simulink model "PID_controller"  (R2013a)
settings: Solver=ode45  StartTime=0.0  StopTime=10.0  RelTol=1e-3
settings Model: Creator=training-it  LastModifiedBy=Pera
settings DataIOCC: SignalLoggingSaveFormat=ModelDataLogs
settings DebuggingCC: MultiTaskDSMMsg=warning  MultiTaskCondExecSysMsg=none  StateNameClashWarn=none  StrictBusMsg=None
settings RTWCC: IncludeERTFirstTime=on

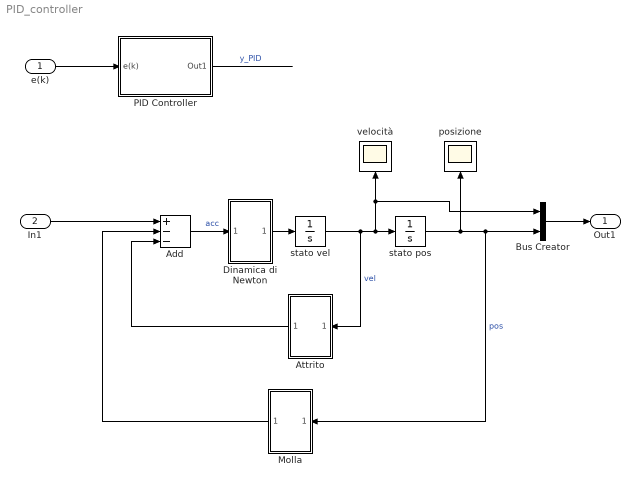
== system PID_controller ==
  e(k) : Inport
  In1 : Inport  Port=2
  Add : Sum  Inputs=+--
  Attrito : Subsystem  mask{c=2}
      mask prompts: c "coeff attrito"
  Bus Creator : BusCreator  Inputs=2
  Dinamica di Newton : Subsystem  mask{m=2}
      mask prompts: m "mass"
  Molla : Subsystem  mask{k=100}
      mask prompts: k "coeff elastico"
  PID Controller : Subsystem  mask{Ts=0.01, kp=0.3, ki=2, kd=0.1}
      mask prompts: Ts "Sample Time"; kp "Guadagno Proporzionale"; ki "Guadagno Integrativo"; kd "Guadagno Derivativo"
      mask init:
      | s1=['kp= ',num2str(kp)];
      | s2=['ki= ',num2str(ki)];
      | s3=['kd= ',num2str(ki)];
      | s=strvcat(s1,s2,s3);  %sto concatenando verticalmente
      mask Display: disp(s)
  posizione : Scope
  stato pos : Integrator  InitialCondition=x0  mask{x0=0}
      mask prompts: x0 "posizione iniziale"
  stato vel : Integrator  mask{v0=0}
      mask prompts: v0 "velocità iniziale"
  velocità : Scope
  Out1 : Outport
  wires:
  e(k)/1 -> PID Controller/1(e(k))
  PID Controller/1(Out1) -> ?  "y_PID"
  stato pos/1 -> Bus Creator/2, Molla/1(In1), posizione/1  "pos"
  Attrito/1(Out1) -> Add/3
  Molla/1(Out1) -> Add/2
  In1/1 -> Add/1
  Add/1 -> Dinamica di Newton/1(In1)  "acc"
  stato vel/1 -> Attrito/1(In1), velocità/1, Bus Creator/1, stato pos/1  "vel"
  Dinamica di Newton/1(Out1) -> stato vel/1
  Bus Creator/1 -> Out1/1

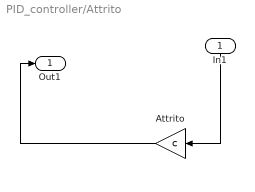
== system PID_controller/Attrito ==
  In1 : Inport
  Attrito : Gain  Gain=c
  Out1 : Outport
  wires:
  Attrito/1 -> Out1/1
  In1/1 -> Attrito/1

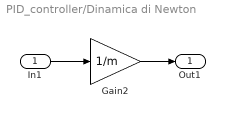
== system PID_controller/Dinamica di Newton ==
  In1 : Inport
  Gain2 : Gain  Gain=1/m
  Out1 : Outport
  wires:
  Gain2/1 -> Out1/1
  In1/1 -> Gain2/1

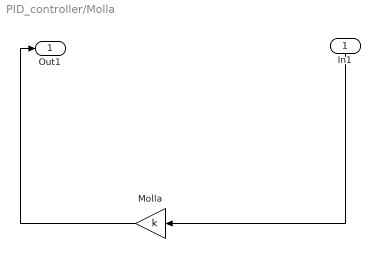
== system PID_controller/Molla ==
  In1 : Inport
  Molla : Gain  Gain=k
  Out1 : Outport
  wires:
  Molla/1 -> Out1/1
  In1/1 -> Molla/1

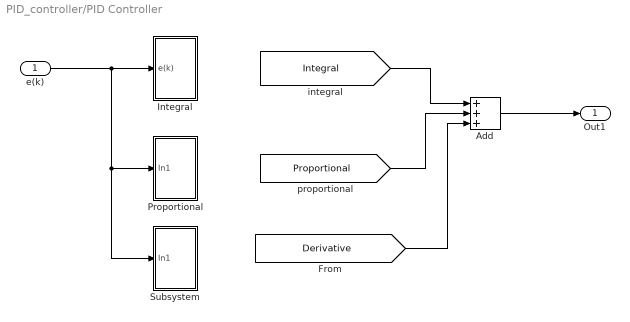
== system PID_controller/PID Controller ==
  e(k) : Inport
  Add : Sum  Inputs=+++
  Integral : Subsystem
  Proportional : Subsystem
  Subsystem : Subsystem
  Out1 : Outport
  wires:
  [Integral] -> Add/1
  Add/1 -> Out1/1
  [Proportional] -> Add/2
  e(k)/1 -> Subsystem/1(In1), Proportional/1(In1), Integral/1(e(k))
  [Derivative] -> Add/3

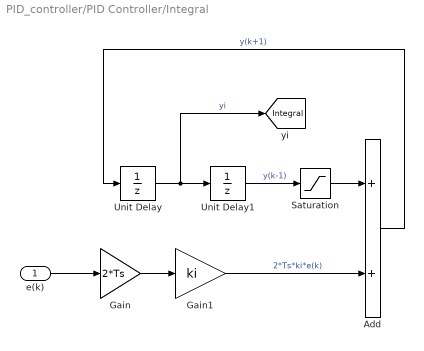
== system PID_controller/PID Controller/Integral ==
  e(k) : Inport
  Add : Sum
  Gain : Gain  Gain=2*Ts
  Gain1 : Gain  Gain=ki
  Saturation : Saturate  UpperLimit=1  LowerLimit=-1
      settings: AttributesFormatString=|
      | %<LowerLimit>
      | %<UpperLimit>
  Unit Delay : UnitDelay  SampleTime=Ts
  Unit Delay1 : UnitDelay  SampleTime=Ts
  tag scope: Integral=global
  wires:
  Gain1/1 -> Add/2  "2*Ts*ki*e(k)"
  Unit Delay/1 -> [Integral], Unit Delay1/1  "yi"
  Gain/1 -> Gain1/1
  Saturation/1 -> Add/1
  Unit Delay1/1 -> Saturation/1  "y(k-1)"
  e(k)/1 -> Gain/1
  Add/1 -> Unit Delay/1  "y(k+1)"

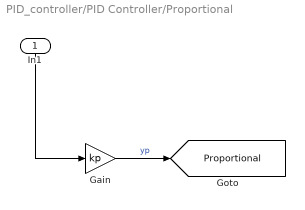
== system PID_controller/PID Controller/Proportional ==
  In1 : Inport
  Gain : Gain  Gain=kp
  tag scope: Proportional=global
  wires:
  Gain/1 -> [Proportional]  "yp"
  In1/1 -> Gain/1

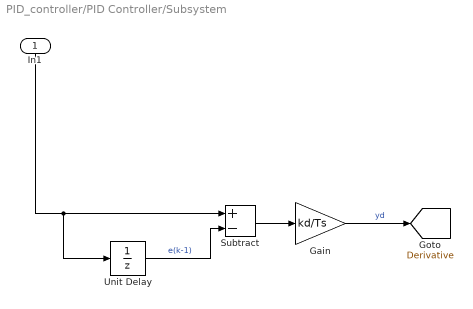
== system PID_controller/PID Controller/Subsystem ==
  In1 : Inport
  Gain : Gain  Gain=kd/Ts
  Subtract : Sum  Inputs=+-
  Unit Delay : UnitDelay  SampleTime=-1
  tag scope: Derivative=global
  wires:
  Unit Delay/1 -> Subtract/2  "e(k-1)"
  Gain/1 -> [Derivative]  "yd"
  Subtract/1 -> Gain/1
  In1/1 -> Unit Delay/1, Subtract/1
